simulink model "Lectura_Sensores"  (R2024b)
settings: Solver=FixedStepAuto  StartTime=0.0  StopTime=inf  FixedStep=0.0001  RelTol=1e-3
undefined symbols (not defined in the file or in its folder): LF
libraries: instrumentseriallib x2
settings Model: Creator=gandr  LastModifiedBy=gandr

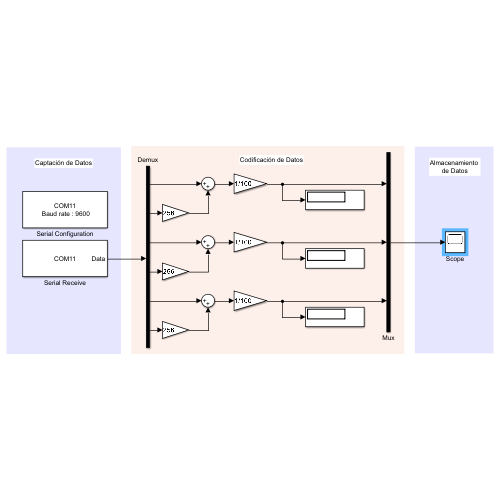
[thumbnail: Simulink's stored preview of the top-level diagram]
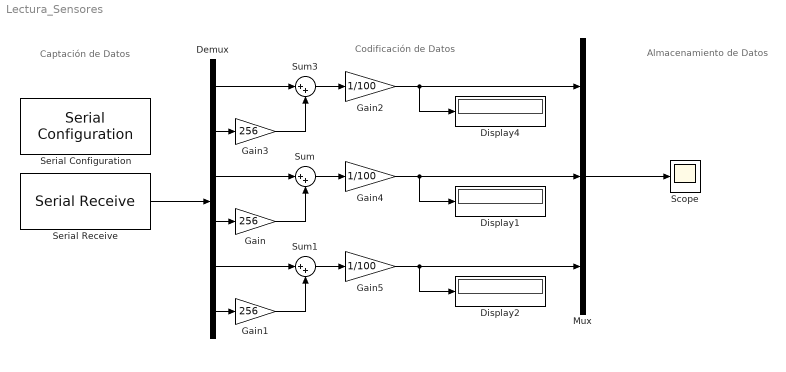
== system Lectura_Sensores ==
  note: Captación de Datos
  note: Almacenamiento
      | de Datos
  note: Codificación de Datos
  Demux : Demux  Outputs=6
  Display1 : Display
  Display2 : Display
  Display4 : Display
  Gain : Gain  Gain=256
  Gain1 : Gain  Gain=256
  Gain2 : Gain  Gain=1/100
  Gain3 : Gain  Gain=256
  Gain4 : Gain  Gain=1/100
  Gain5 : Gain  Gain=1/100
  Mux : Mux  Inputs=3
  Scope : Scope
  Serial Configuration : instrumentseriallib/Serial Configuration  Priority=-200000  PortSel=COM11  Port=COM11  ComPort=COM11  BaudRate=9600  DataBits=8  Parity=none  StopBits=1  ByteOrder=little-endian  FlowControl=none  Timeout=10  SimulateUsing=Interpreted execution  BlockInModel=on  aMode=1
  Serial Receive : instrumentseriallib/Serial Receive  Priority=1  PortSel=COM11  Port=COM11  ComPort=COM11  DataType=uint8  SaveDataType=uint8  ToggleHeader=on  Header='A'  ToggleDataSize=on  DataSize=6  ToggleTerminator=on  Terminator=LF ('\n')  CustomTerminator=[]  InputFormat=Column major  EnableBlockingMode=on  ActionDataUnavailable=Output last received value  ActionWhenDataUnavailable=Output last received value  CustomValue=0  SampleTime=0.01  SimulateUsing=Interpreted execution  BlockInModel=on  aMode=1
  Sum : Sum  Inputs=|++
  Sum1 : Sum  Inputs=|++
  Sum3 : Sum  Inputs=|++
  wires:
  Demux/2 -> Gain3/1
  Gain1/1 -> Sum1/2
  Demux/3 -> Sum/1
  Gain/1 -> Sum/2
  Demux/6 -> Gain1/1
  Serial Receive/1 -> Demux/1
  Demux/5 -> Sum1/1
  Gain3/1 -> Sum3/2
  Sum/1 -> Gain4/1
  Sum3/1 -> Gain2/1
  Mux/1 -> Scope/1
  Demux/1 -> Sum3/1
  Sum1/1 -> Gain5/1
  Demux/4 -> Gain/1
  Gain2/1 -> Mux/1, Display4/1
  Gain4/1 -> Mux/2, Display1/1
  Gain5/1 -> Mux/3, Display2/1
